simulink model "ysw11_8"  (R2014a)
settings: Solver=ode45  StartTime=0.0  StopTime=10.0  RelTol=1e-3
libraries: commanapbnd3 x1
settings Model: Creator=ii  LastModifiedBy=ii
settings SolverCC: ZeroCrossAlgorithm=Adaptive
settings DebuggingCC: UnderspecifiedInitializationDetection=Classic

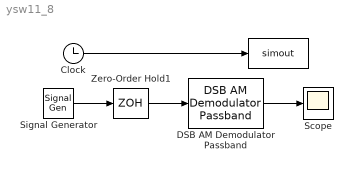
== system ysw11_8 ==
  "  " : ToWorkspace  VariableName=simout  SampleTime=-1
  Clock : Clock
  DSB AM Demodulator Passband : commanapbnd3/DSB AM Demodulator Passband  Fc=300  Ph=0  method=Butterworth  n=8  cf=0.1  Rp=0.1  Rs=50  Offset=1
  Scope : Scope
  Signal Generator : SignalGenerator  Frequency=700  Units=rad/sec
  Zero-Order Hold1 : ZeroOrderHold
  wires:
  Signal Generator/1 -> Zero-Order Hold1/1
  Clock/1 -> "  "/1
  DSB AM Demodulator Passband/1 -> Scope/1
  Zero-Order Hold1/1 -> DSB AM Demodulator Passband/1
